simulink model "FilterVerification"  (R2019b)
settings: Solver=VariableStepAuto  StartTime=0.0  StopTime=10.0  MaxStep=0.001  RelTol=1e-3
settings Model: Creator=ip  LastModifiedBy=ip

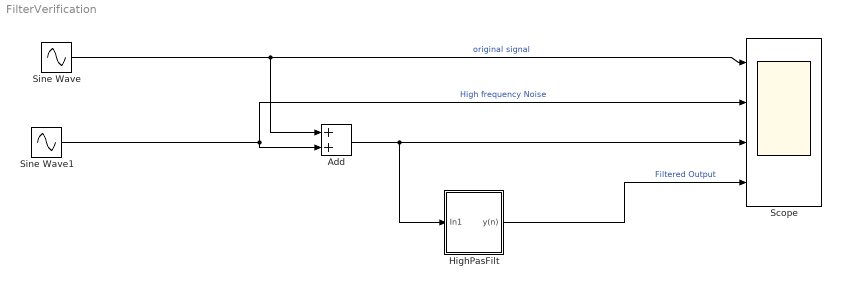
== system FilterVerification ==
  Add : Sum
  HighPasFilt : Subsystem
  Scope : Scope  NumInputPorts=4
  Sine Wave : Sin  Amplitude=50  Frequency=1256  SampleTime=0
  Sine Wave1 : Sin  Frequency=125  SampleTime=0
  wires:
  Sine Wave/1 -> Add/1, Scope/1  "original signal"
  HighPasFilt/1(y(n)) -> Scope/4  "Filtered Output"
  Sine Wave1/1 -> Add/2, Scope/2  "High frequency Noise"
  Add/1 -> HighPasFilt/1(In1), Scope/3

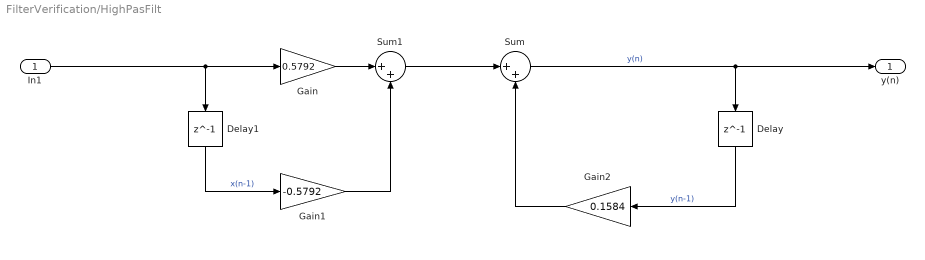
== system FilterVerification/HighPasFilt ==
  In1 : Inport
  Delay : Delay  DelayLength=1
  Delay1 : Delay  DelayLength=1
  Gain : Gain  Gain=0.5792
  Gain1 : Gain  Gain=-0.5792
  Gain2 : Gain  Gain=0.1584
  Sum : Sum  Inputs=|++
  Sum1 : Sum  Inputs=|++
  y(n) : Outport
  wires:
  Sum1/1 -> Sum/1
  Sum/1 -> y(n)/1, Delay/1  "y(n)"
  In1/1 -> Gain/1, Delay1/1
  Gain1/1 -> Sum1/2
  Delay/1 -> Gain2/1  "y(n-1)"
  Gain/1 -> Sum1/1
  Delay1/1 -> Gain1/1  "x(n-1)"
  Gain2/1 -> Sum/2
